simulink model "batch_events_3_supervisors"  (R2021b)
settings: Solver=ode4  StartTime=0.0  StopTime=inf  FixedStep=0.001  RelTol=1e-3  EnableMultiTasking=on
model workspace (MATLAB code in the model file):
  | % Add the class folders into the path.
  | addpath src/model
  | addpath src/utils
  | 
  | %% Loading data from files.
  | % Data for supervisor 1.
  | utils1 = StateMachineUtils;
  | 
  | % From TCT: Load all events' number.
  | utils1 = utils1.loadEventsInAds('resources/tct/ALLEVENT.ADS');
  | 
  | % From TCT: Disabled events in each state.
  | utils1 = utils1.loadDisabledEventsInPdt('resources/tct/supervisor1/DATA_SIMSUP1_MG1.PDT');
  | 
  | % From TCT: Transition matrix.
  | utils1 = utils1.loadTransitionsInAds('resources/tct/supervisor1/SIMSUP1_MG1.ADS');
  | 
  | % Parameters for the block.
  | encodedStates1 = StateEncoder.encode(utils1.statesArray);
  | 
  | transitions1 = utils1.transitions;
  | 
  | allEvents1 = utils1.eventsArray;
  | 
  | % Data for supervisor 2.
  | utils2 = StateMachineUtils;
  | 
  | % From TCT: Load all events' number.
  | utils2 = utils2.loadEventsInAds('resources/tct/ALLEVENT.ADS');
  | 
  | % From TCT: Disabled events in each state.
  | utils2 = utils2.loadDisabledEventsInPdt('resources/tct/supervisor2/DATA_SIMSUP2_MG1.PDT');
  | 
  | % From TCT: Transition matrix.
  | utils2 = utils2.loadTransitionsInAds('resources/tct/supervisor2/SIMSUP2_MG1.ADS');
  | 
  | % Parameters for the block.
  | encodedStates2 = StateEncoder.encode(utils2.statesArray);
  | 
  | transitions2 = utils2.transitions;
  | 
  | allEvents2 = utils2.eventsArray;
  | 
  | % Data for supervisor 3.
  | utils3 = StateMachineUtils;
  | 
  | % From TCT: Load all events' number.
  | utils3 = utils3.loadEventsInAds('resources/tct/ALLEVENT.ADS');
  | 
  | % From TCT: Disabled events in each state.
  | utils3 = utils3.loadDisabledEventsInPdt('resources/tct/supervisor3/DATA_SIMSUP3_MG1.PDT');
  | 
  | % From TCT: Transition matrix.
  | utils3 = utils3.loadTransitionsInAds('resources/tct/supervisor3/SIMSUP3_MG1.ADS');
  | 
  | % Parameters for the block.
  | encodedStates3 = StateEncoder.encode(utils3.statesArray);
  | 
  | transitions3 = utils3.transitions;
  | 
  | allEvents3 = utils3.eventsArray;
libraries: rtlab x2
Description:
  | Model of a simple control system for use iin training.
settings Model: Creator=Paul Baracos  LastModifiedBy=andrerangel
settings SolverCC: AlgebraicLoopSolver=TrustRegion
settings DataIOCC: LimitDataPoints=on  SaveFormat=Array  SignalLoggingSaveFormat=ModelDataLogs  SaveOutput=off  SaveTime=off  ReturnWorkspaceOutputs=off  SignalLoggingName=sigsOut
settings OptimizationCC: BlockReduction=off  BooleanDataType=off  OptimizeBlockIOStorage=off  BufferReuse=off  ExpressionFolding=off  LocalBlockOutputs=off  InitFltsAndDblsToZero=on  LifeSpan=inf
settings DebuggingCC: SaveWithParameterizedLinksMsg=none  UnderspecifiedInitializationDetection=Classic  MergeDetectMultiDrivingBlocksExec=none  SignalResolutionControl=TryResolveAllWithWarning  MultiTaskDSMMsg=warning  MultiTaskCondExecSysMsg=none  FcnCallInpInsideContextMsg=warning  SFUnexpectedBacktrackingDiag=warning  SFNoUnconditionalDefaultTransitionDiag=warning  SFExecutionAtInitializationDiag=none  SFMachineParentedDataDiag=warning  ArithmeticOperatorsInVariantConditions=warning
settings HardwareCC: ProdBitPerPointer=32  ProdBitPerSizeT=32  ProdBitPerPtrDiffT=32  ProdLargestAtomicFloat=None  ProdIntDivRoundTo=Undefined  ProdEndianess=Unspecified  ProdWordSize=32  ProdHWDeviceType=32-bit Generic  TargetUnknown=on
settings ModelReferenceCC: PropagateSignalLabelsOutOfModel=off
settings SFSimCC: SimUseLocalCustomCode=off  CustomCodeUndefinedFunction=UseInterfaceOnly
settings RTWCC: RTWUseLocalCustomCode=off
settings CodeAppCC: StateflowObjectComments=on
settings GRTTargetCC: TargetFcnLib=ansi_tfl_tmw.mat  TargetLangStandard=C89/C90 (ANSI)  CombineOutputUpdateFcns=off  GRTInterface=on
settings ConfigComp: CovMetricSettings=dw  CovSaveCumulativeToWorkspaceVar=on  CovSaveSingleToWorkspaceVar=on  CovExternalEMLEnable=off

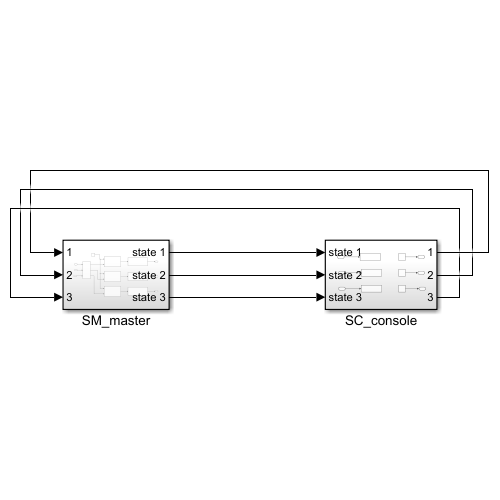
[thumbnail: Simulink's stored preview of the top-level diagram]
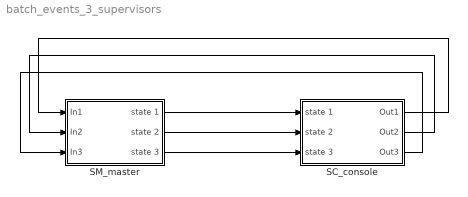
== system batch_events_3_supervisors ==
  SC_console : Subsystem
  SM_master : Subsystem
  wires:
  SM_master/1(state 1) -> SC_console/1(state 1)
  SM_master/2(state 2) -> SC_console/2(state 2)
  SM_master/3(state 3) -> SC_console/3(state 3)
  SC_console/1(Out1) -> SM_master/1(In1)
  SC_console/2(Out2) -> SM_master/2(In2)
  SC_console/3(Out3) -> SM_master/3(In3)

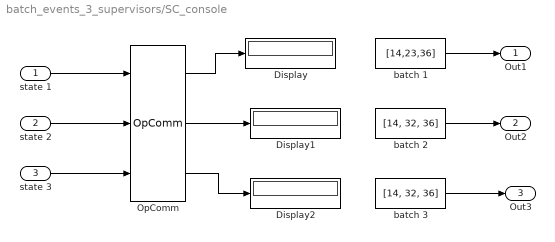
== system batch_events_3_supervisors/SC_console ==
  state 1 : Inport
  state 2 : Inport  Port=2
  state 3 : Inport  Port=3
  Display : Display
  Display1 : Display
  Display2 : Display
  OpComm : rtlab/OpComm  nbport=3  groupe_acq=1  subsys_rate=0  st=0  Synchronization=on  Interpolation=on  Threshold=1.0  Missed_Data=off  Sim_Time=off  Samples=off  dynSigOut=off  from_console=0  warning_done=off  writeOpCommFile=off  Offset=off
      settings: SourceProductName=RT-LAB
  batch 1 : Constant  Value=[14,23,36]
  batch 2 : Constant  Value=[14, 32, 36]
  batch 3 : Constant  Value=[14, 32, 36]
  Out1 : Outport
  Out2 : Outport  Port=2
  Out3 : Outport  Port=3
  wires:
  batch 1/1 -> Out1/1
  batch 3/1 -> Out3/1
  batch 2/1 -> Out2/1
  state 1/1 -> OpComm/1
  state 2/1 -> OpComm/2
  state 3/1 -> OpComm/3
  OpComm/1 -> Display/1
  OpComm/2 -> Display1/1
  OpComm/3 -> Display2/1

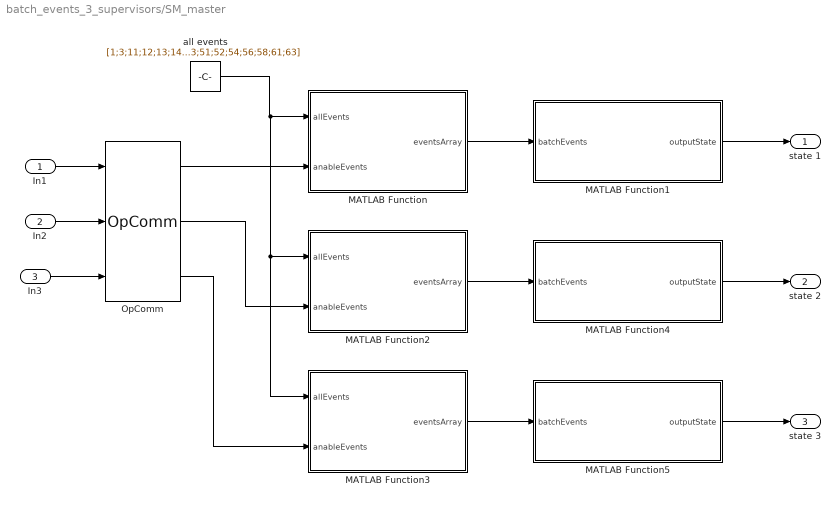
== system batch_events_3_supervisors/SM_master ==
  In1 : Inport
  In2 : Inport  Port=2
  In3 : Inport  Port=3
  MATLAB Function : MATLAB Function  TreatAsAtomicUnit=on
  MATLAB Function1 : MATLAB Function  TreatAsAtomicUnit=on
  MATLAB Function2 : MATLAB Function  TreatAsAtomicUnit=on
  MATLAB Function3 : MATLAB Function  TreatAsAtomicUnit=on
  MATLAB Function4 : MATLAB Function  TreatAsAtomicUnit=on
  MATLAB Function5 : MATLAB Function  TreatAsAtomicUnit=on
  OpComm : rtlab/OpComm  nbport=3  groupe_acq=1  subsys_rate=0  st=0  Synchronization=on  Interpolation=on  Threshold=1.0  Missed_Data=off  Sim_Time=off  Samples=off  dynSigOut=off  from_console=1  warning_done=off  writeOpCommFile=off  Offset=off
      settings: SourceProductName=RT-LAB
  all events : Constant  Value=[1;3;11;12;13;14;16;21;23;25;27;31;32;33;34;36;41;43;51;52;54;56;58;61;63]
  state 1 : Outport
  state 2 : Outport  Port=2
  state 3 : Outport  Port=3
  wires:
  In1/1 -> OpComm/1
  OpComm/1 -> MATLAB Function/2(anableEvents)
  MATLAB Function/1(eventsArray) -> MATLAB Function1/1(batchEvents)
  MATLAB Function1/1(outputState) -> state 1/1
  all events/1 -> MATLAB Function3/1(allEvents), MATLAB Function2/1(allEvents), MATLAB Function/1(allEvents)
  In2/1 -> OpComm/2
  In3/1 -> OpComm/3
  OpComm/2 -> MATLAB Function2/2(anableEvents)
  OpComm/3 -> MATLAB Function3/2(anableEvents)
  MATLAB Function2/1(eventsArray) -> MATLAB Function4/1(batchEvents)
  MATLAB Function3/1(eventsArray) -> MATLAB Function5/1(batchEvents)
  MATLAB Function5/1(outputState) -> state 3/1
  MATLAB Function4/1(outputState) -> state 2/1

== matlab function batch_events_3_supervisors/SM_master/MATLAB Function1 ==
  data: batchEvents input; outputState output; encodedStates1 parameter; transitions1 parameter; allEvents1 parameter
function outputState  = stateMachine1(batchEvents, encodedStates1, transitions1, allEvents1)
% State Machine with parameters from files.
% Receives a batch of events and process one event at time, starting with
% the event of index 1.
% batchEvents: array with 0s and 1s where 1 is the enabled event while 0,
% is disabled event;
% allEvents: numbers of the events;
% transitions: matrix of transitions;
% encodedStates: Encoded states array to be decoded before the pass it to
% StateMachines as an argument.

% Initialize a persistent object. Its value will not be erased as this
% block finishes.
persistent stateMachine

% Assign the persistent object to the StateMachine class with data passed
% as parameters.
if (isempty(stateMachine))
    statesArray = StateEncoder.decode(encodedStates1);                        
    stateMachine = StateMachine(statesArray, transitions1, allEvents1);
end

anabledEvents = allEvents1(logical(batchEvents));

% loop through an array of events:
for i=1:length(anabledEvents)
    stateMachine.inputEvent = anabledEvents(i);
end
outputState = double(stateMachine.currentState.number);

== matlab function batch_events_3_supervisors/SM_master/MATLAB Function ==
  data: allEvents input; eventsArray output; anableEvents input
function eventsArray = eventsGenerator(allEvents, anableEvents)

[~, indexes] = ismember(anableEvents, allEvents);

eventsArray = zeros(length(allEvents), 1);

eventsArray(indexes) = 1;

== matlab function batch_events_3_supervisors/SM_master/MATLAB Function2 ==
  data: allEvents input; eventsArray output; anableEvents input
function eventsArray = eventsGenerator(allEvents, anableEvents)

[~, indexes] = ismember(anableEvents, allEvents);

eventsArray = zeros(length(allEvents), 1);

eventsArray(indexes) = 1;

== matlab function batch_events_3_supervisors/SM_master/MATLAB Function3 ==
  data: allEvents input; eventsArray output; anableEvents input
function eventsArray = eventsGenerator(allEvents, anableEvents)

[~, indexes] = ismember(anableEvents, allEvents);

eventsArray = zeros(length(allEvents), 1);

eventsArray(indexes) = 1;

== matlab function batch_events_3_supervisors/SM_master/MATLAB Function4 ==
  data: batchEvents input; outputState output; encodedStates2 parameter; transitions2 parameter; allEvents2 parameter
function outputState  = stateMachine2(batchEvents, encodedStates2, transitions2, allEvents2)
% State Machine with parameters from files.
% Receives a batch of events and process one event at time, starting with
% the event of index 1.
% batchEvents: array with 0s and 1s where 1 is the enabled event while 0,
% is disabled event;
% allEvents: numbers of the events;
% transitions: matrix of transitions;
% encodedStates: Encoded states array to be decoded before the pass it to
% StateMachines as an argument.

% Initialize a persistent object. Its value will not be erased as this
% block finishes.
persistent stateMachine

% Assign the persistent object to the StateMachine class with data passed
% as parameters.
if (isempty(stateMachine))
    statesArray = StateEncoder.decode(encodedStates2);                        
    stateMachine = StateMachine(statesArray, transitions2, allEvents2);
end

anabledEvents = allEvents2(logical(batchEvents));

% loop through an array of events:
for i=1:length(anabledEvents)
    stateMachine.inputEvent = anabledEvents(i);
end
outputState = double(stateMachine.currentState.number);

== matlab function batch_events_3_supervisors/SM_master/MATLAB Function5 ==
  data: batchEvents input; outputState output; encodedStates3 parameter; transitions3 parameter; allEvents3 parameter
function outputState  = stateMachine3(batchEvents, encodedStates3, transitions3, allEvents3)
% State Machine with parameters from files.
% Receives a batch of events and process one event at time, starting with
% the event of index 1.
% batchEvents: array with 0s and 1s where 1 is the enabled event while 0,
% is disabled event;
% allEvents: numbers of the events;
% transitions: matrix of transitions;
% encodedStates: Encoded states array to be decoded before the pass it to
% StateMachines as an argument.

% Initialize a persistent object. Its value will not be erased as this
% block finishes.
persistent stateMachine

% Assign the persistent object to the StateMachine class with data passed
% as parameters.
if (isempty(stateMachine))
    statesArray = StateEncoder.decode(encodedStates3);                        
    stateMachine = StateMachine(statesArray, transitions3, allEvents3);
end

anabledEvents = allEvents3(logical(batchEvents));

% loop through an array of events:
for i=1:length(anabledEvents)
    stateMachine.inputEvent = anabledEvents(i);
end
outputState = double(stateMachine.currentState.number);
